simulink library "marlo_lib_v01"  (Simulink 8.1)
settings: Solver=ode45  StartTime=0.0  StopTime=10.0  RelTol=1e-3
undefined symbols (not defined in the file or in its folder): A_deriv_encoder, A_deriv_IMU, ANOMALY_INIT, B_deriv_encoder, B_deriv_IMU, C_deriv_encoder, C_deriv_IMU, CalibrationParams, Com1, D_deriv_encoder, D_deriv_IMU, Dt_deriv_encoder, Dt_deriv_IMU, EncoderAngleLimits, EncoderThreshold, IMUAngleLimits, IMUParams, IMUThreshold, KVHOrientationCal, m_XR17D15x, MAX_ANOMALY, MotorParams, none, standard, x0_deriv_encoder, x0_deriv_IMU, XOFF, XON
libraries: xpcethercatlib x307, speedgoatlib x26, xpcseriallib x15, simulink x8, marlo_lib_v01 x6, dspswit3 x2, xpclib x1
(part 5 of 6)

== system marlo_lib_v01/DAQ_WITH_SAFETY_IMU/DAQ/SerialIMU/TPMC466 ==
  In1 : Inport
  In2 : Inport  Port=2
  In3 : Inport  Port=3
  In4 : Inport  Port=4
  Board Setup : speedgoatlib/IO503/TEWS TPMC466 Internal blocks/Board Setup  irqnum=9  slot=brdslot
  "Enable TX " : speedgoatlib/IO503/TEWS TPMC466 Internal blocks/Enable TX   port=1  slot=brdslot
  Enable TX 1 : speedgoatlib/IO503/TEWS TPMC466 Internal blocks/Enable TX   port=2  slot=brdslot
  Enable TX 2 : speedgoatlib/IO503/TEWS TPMC466 Internal blocks/Enable TX   port=3  slot=brdslot
  Enable TX 3 : speedgoatlib/IO503/TEWS TPMC466 Internal blocks/Enable TX   port=4  slot=brdslot
  FIFO write 1 : xpcseriallib/FIFO write   size=1024  inputtype=8 bit uint null terminated  present=on  sampletime=-1  id=XMT channel 1, IRQ 9
  FIFO write 2 : xpcseriallib/FIFO write   size=1024  inputtype=8 bit uint null terminated  present=on  sampletime=-1  id=XMT channel 2, IRQ 9
  FIFO write 3 : xpcseriallib/FIFO write   size=1024  inputtype=8 bit uint null terminated  present=on  sampletime=-1  id=XMT channel 3, IRQ 9
  FIFO write 4 : xpcseriallib/FIFO write   size=1024  inputtype=8 bit uint null terminated  present=on  sampletime=-1  id=XMT channel 4, IRQ 9
  IRQ Source : xpclib/Asynchronous Event/IRQ Source  irqNo=9  preempt=off  b_type=None/Other  slot=brdslot
  RS232 ISR : Subsystem  TreatAsAtomicUnit=on  mask(RS232 ISR){slot=brdslot}
      mask help:
      | PMC521
      | Acromag
      | Interrupt Service Routine
      mask init:
      | subslot = slot;
      mask Display:
      | disp('PMC521\nAcromag\nISR');
      | port_label('input', 1, 'XMT1');
      | port_label('input', 2, 'XMT2');
      | port_label('input', 3, 'XMT3');
      | port_label('input', 4, 'XMT4');
      | port_label('input', 5, 'XMT5');
      | port_label('input', 6, 'XMT6');
      | port_label('input', 7, 'XMT7');
      | port_label('input', 8, 'XMT8');
      | port_label('output', 1, 'RCV1');
      | port_label('output', 2, 'RCV2');
      | port_label('output', 3, 'RCV3');
      | port_label('output', 4, 'RCV4');
      | port_label('output', 5, 'RCV5');
      | port_label('output', 6, 'RCV6');
      | port_label('output', 7, 'RCV7');
      | port_label('output', 8, 'RCV8');
  Rate Transition{,2,4..5} (4 alike) : RateTransition  Integrity=off  Deterministic=off
  Rate Transition{1,3,6..7} (4 alike) : RateTransition  Integrity=off  Deterministic=off  OutPortSampleTime=0
  Setup1 : speedgoatlib/IO503/TEWS TPMC466 Internal blocks/Setup   port=1  transceiver=RS422  standard=on  baudrate=921600  bauddivisor=1  mode8x=16x (standard)  prescale=off  width=8  nstop=1  parity=None  rlevel=quarter full (16)  ctsmode=none  xonoff=none  xon=17  xoff=19  rs485mode=off  rs485delay=1  slot=brdslot
  Setup2 : speedgoatlib/IO503/TEWS TPMC466 Internal blocks/Setup   port=2  transceiver=RS485 half-duplex  standard=on  baudrate=2764800  bauddivisor=1  mode8x=16x (standard)  prescale=off  width=8  nstop=1  parity=None  rlevel=quarter full (16)  ctsmode=none  xonoff=XON/XOFF  xon=17  xoff=19  rs485mode=on  rs485delay=1  slot=brdslot
  Setup3 : speedgoatlib/IO503/TEWS TPMC466 Internal blocks/Setup   port=3  transceiver=RS485 half-duplex  standard=on  baudrate=115200  bauddivisor=1  mode8x=16x (standard)  prescale=off  width=8  nstop=1  parity=None  rlevel=half full (32)  ctsmode=none  xonoff=none  xon=17  xoff=19  rs485mode=off  rs485delay=0  slot=brdslot
  Setup4 : speedgoatlib/IO503/TEWS TPMC466 Internal blocks/Setup   port=4  transceiver=RS485 half-duplex  standard=on  baudrate=115200  bauddivisor=1  mode8x=16x (standard)  prescale=off  width=8  nstop=1  parity=None  rlevel=half full (32)  ctsmode=none  xonoff=none  xon=17  xoff=19  rs485mode=off  rs485delay=0  slot=brdslot
  Out1 : Outport
  Out2 : Outport  Port=2
  Out3 : Outport  Port=3
  Out4 : Outport  Port=4
  wires:
  FIFO write 2/2 -> Enable TX 1/1
  In2/1 -> FIFO write 2/1
  FIFO write 2/1 -> Rate Transition2/1
  In1/1 -> FIFO write 1/1
  FIFO write 1/1 -> Rate Transition/1
  RS232 ISR/2(Recv 2) -> Rate Transition3/1
  RS232 ISR/1(Recv 1) -> Rate Transition1/1
  IRQ Source/1 -> RS232 ISR/Trigger
  FIFO write 1/2 -> "Enable TX "/1
  Rate Transition2/1 -> RS232 ISR/2(Xmt 2)
  Rate Transition/1 -> RS232 ISR/1(Xmt 1)
  Rate Transition3/1 -> Out2/1
  Rate Transition1/1 -> Out1/1
  FIFO write 3/2 -> Enable TX 2/1
  In3/1 -> FIFO write 3/1
  FIFO write 3/1 -> Rate Transition4/1
  FIFO write 4/2 -> Enable TX 3/1
  In4/1 -> FIFO write 4/1
  FIFO write 4/1 -> Rate Transition5/1
  Rate Transition4/1 -> RS232 ISR/3(Xmt 3)
  Rate Transition5/1 -> RS232 ISR/4(Xmt 4)
  Rate Transition6/1 -> Out3/1
  Rate Transition7/1 -> Out4/1
  RS232 ISR/3(Recv 3) -> Rate Transition6/1
  RS232 ISR/4(Recv 4) -> Rate Transition7/1

== system marlo_lib_v01/DAQ_WITH_SAFETY_IMU/DAQ/SerialIMU/UpdateOrientation ==
  FIFO : Inport
  Reset : Inport  Port=2
  Zero : Inport  Port=3
  Assignment : Assignment  IndexOptions=Index vector (port)  Indices=1  OutputSizes=1
  Compare To Constant1 : simulink/Logic and Bit Operations/Compare To Constant  relop===  const=1  OutDataTypeStr=uint8
  EstimateOrientation : MATLAB Function  TreatAsAtomicUnit=on
  "FIFO bin read " : xpcseriallib/FIFO bin read   header={char([254 129 255 85])}  lengths=[36]  hold=Zero output if no new data  enable=off  maxsize=36  outputtype=8 bit uint null terminated  sampletime=-1
  For Iterator : ForIterator
  MATLAB Function : MATLAB Function  TreatAsAtomicUnit=on
  Product : Product  RndMeth=Zero
  Unit Delay : UnitDelay  InitialCondition=[0; 0; 0]  SampleTime=-1
  Unit Delay1 : UnitDelay  InitialCondition=zeros(3,3)  SampleTime=-1
  Unit Delay2 : UnitDelay  InitialCondition=[0; 0; 0]  SampleTime=-1
  Unit Delay3 : UnitDelay  SampleTime=-1
  Rk : Outport  InitialOutput=zeros(3,3)
  wk : Outport  Port=2  InitialOutput=zeros(3,1)
  DeltaAngle : Outport  Port=3  InitialOutput=zeros(3,1)
  Acceleration : Outport  Port=4  InitialOutput=zeros(3,1)
  Status : Outport  Port=5  InitialOutput=0
  Sequence : Outport  Port=6  InitialOutput=[0; 0; 0; 0; 0]
  Temperature : Outport  Port=7  InitialOutput=0
  Valid : Outport  Port=8  InitialOutput=0
  wires:
  Unit Delay2/1 -> EstimateOrientation/7(wkm1)
  EstimateOrientation/2(wk) -> Unit Delay2/1, wk/1
  For Iterator/1 -> [Iter]
  Zero/1 -> Assignment/1
  Assignment/1 -> Sequence/1
  [Iter] -> Assignment/3
  "FIFO bin read "/1 -> MATLAB Function/1(P)
  Reset/1 -> [Reset]
  Unit Delay3/1 -> EstimateOrientation/9(Seqkm1)
  EstimateOrientation/4(Seqk) -> Unit Delay3/1
  FIFO/1 -> "FIFO bin read "/1
  Compare To Constant1/1 -> Product/2
  Product/1 -> EstimateOrientation/3(Status)
  [Reset] -> EstimateOrientation/5(Reset)
  Unit Delay1/1 -> EstimateOrientation/6(Rkm1)
  EstimateOrientation/1(Rk) -> Unit Delay1/1, Rk/1
  Unit Delay/1 -> EstimateOrientation/8(Akm1)
  EstimateOrientation/3(Ak) -> Unit Delay/1
  MATLAB Function/6(Valid) -> Compare To Constant1/1, Valid/1
  MATLAB Function/5(Temperature) -> Temperature/1
  MATLAB Function/4(Sequence) -> EstimateOrientation/4(Sequence), Assignment/2
  MATLAB Function/3(Status) -> Product/1, Status/1
  MATLAB Function/1(Rotation) -> EstimateOrientation/1(DeltaAngle), DeltaAngle/1
  MATLAB Function/2(Acceleration) -> EstimateOrientation/2(Acceleration), Acceleration/1

== system marlo_lib_v01/DAQ_WITH_SAFETY_IMU/DAQ/SerialIMU/TPMC466/RS232 ISR ==
  Xmt 1 : Inport
  Xmt 2 : Inport  Port=2
  Xmt 3 : Inport  Port=3
  Xmt 4 : Inport  Port=4
  function : TriggerPort  TriggerType=function-call
  While Iterator Subsystem : Subsystem  TreatAsAtomicUnit=on
  Recv 1 : Outport  SourceOfInitialOutputValue=Input signal
  Recv 2 : Outport  Port=2  SourceOfInitialOutputValue=Input signal
  Recv 3 : Outport  Port=3  SourceOfInitialOutputValue=Input signal
  Recv 4 : Outport  Port=4  SourceOfInitialOutputValue=Input signal
  wires:
  Xmt 1/1 -> While Iterator Subsystem/1(Xmt 1)
  Xmt 2/1 -> While Iterator Subsystem/2(Xmt 2)
  While Iterator Subsystem/1(Recv 1) -> Recv 1/1
  While Iterator Subsystem/2(Recv 2) -> Recv 2/1
  Xmt 3/1 -> While Iterator Subsystem/3(Xmt 3)
  Xmt 4/1 -> While Iterator Subsystem/4(Xmt 4)
  While Iterator Subsystem/3(Recv 3) -> Recv 3/1
  While Iterator Subsystem/4(Recv 4) -> Recv 4/1

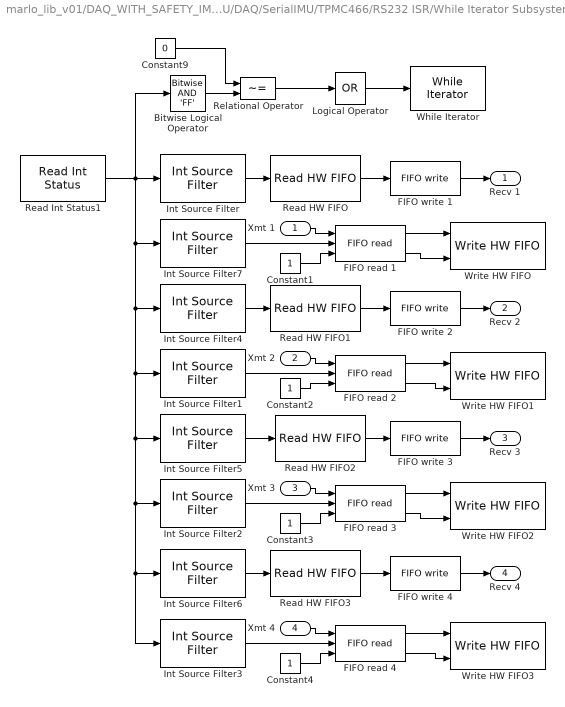
== system marlo_lib_v01/DAQ_WITH_SAFETY_IMU/DAQ/SerialIMU/TPMC466/RS232 ISR/While Iterator Subsystem ==
  Xmt 1 : Inport
  Xmt 2 : Inport  Port=2
  Xmt 3 : Inport  Port=3
  Xmt 4 : Inport  Port=4
  Bitwise Logical Operator : simulink/Logic and Bit Operations/Bitwise Operator  logicop=AND  UseBitMask=on  BitMask='FF'  BitMaskRealWorld=Stored Integer
  Constant{1..4} (4 alike) : Constant  OutDataTypeStr=uint32
  Constant9 : Constant  Value=0  OutDataTypeStr=uint32
  FIFO read {1..4} (4 alike) : xpcseriallib/FIFO read   maxsize=60  minsize=1  usedelimiter=off  delimiter=13  outputtype=count+32 bit uint  enable=on  enableout=on  sampletime=-1
  FIFO write 1 : xpcseriallib/FIFO write   size=1024  inputtype=count+32 bit uint  present=off  sampletime=-1  id=RCV channel 1, IRQ 9
  FIFO write 2 : xpcseriallib/FIFO write   size=1024  inputtype=count+32 bit uint  present=off  sampletime=-1  id=RCV channel 2, IRQ 9
  FIFO write 3 : xpcseriallib/FIFO write   size=1024  inputtype=count+32 bit uint  present=off  sampletime=-1  id=RCV channel 3, IRQ 9
  FIFO write 4 : xpcseriallib/FIFO write   size=1024  inputtype=count+32 bit uint  present=off  sampletime=-1  id=RCV channel 4, IRQ 9
  Int Source Filter : speedgoatlib/IO503/TEWS TPMC466 Internal blocks/Int Source Filter  port=1  value=Receive data
  Int Source Filter1 : speedgoatlib/IO503/TEWS TPMC466 Internal blocks/Int Source Filter  port=2  value=Transmitter empty
  Int Source Filter2 : speedgoatlib/IO503/TEWS TPMC466 Internal blocks/Int Source Filter  port=3  value=Transmitter empty
  Int Source Filter3 : speedgoatlib/IO503/TEWS TPMC466 Internal blocks/Int Source Filter  port=4  value=Transmitter empty
  Int Source Filter4 : speedgoatlib/IO503/TEWS TPMC466 Internal blocks/Int Source Filter  port=2  value=Receive data
  Int Source Filter5 : speedgoatlib/IO503/TEWS TPMC466 Internal blocks/Int Source Filter  port=3  value=Receive data
  Int Source Filter6 : speedgoatlib/IO503/TEWS TPMC466 Internal blocks/Int Source Filter  port=4  value=Receive data
  Int Source Filter7 : speedgoatlib/IO503/TEWS TPMC466 Internal blocks/Int Source Filter  port=1  value=Transmitter empty
  Logical Operator : Logic  Operator=OR  Inputs=1  AllPortsSameDT=off
  Read HW FIFO : speedgoatlib/IO503/TEWS TPMC466 Internal blocks/Read HW FIFO  port=1  flush=on  slot=subslot
  Read HW FIFO1 : speedgoatlib/IO503/TEWS TPMC466 Internal blocks/Read HW FIFO  port=2  flush=on  slot=subslot
  Read HW FIFO2 : speedgoatlib/IO503/TEWS TPMC466 Internal blocks/Read HW FIFO  port=3  flush=on  slot=subslot
  Read HW FIFO3 : speedgoatlib/IO503/TEWS TPMC466 Internal blocks/Read HW FIFO  port=4  flush=on  slot=subslot
  Read Int Status1 : speedgoatlib/IO503/TEWS TPMC466 Internal blocks/Read Int Status  slot=subslot
  Relational Operator : RelationalOperator  Operator=~=
  While Iterator : WhileIterator  MaxIters=65  WhileBlockType=do-while
  Write HW FIFO : speedgoatlib/IO503/TEWS TPMC466 Internal blocks/Write HW FIFO  port=1  slot=subslot
  Write HW FIFO1 : speedgoatlib/IO503/TEWS TPMC466 Internal blocks/Write HW FIFO  port=2  slot=subslot
  Write HW FIFO2 : speedgoatlib/IO503/TEWS TPMC466 Internal blocks/Write HW FIFO  port=3  slot=subslot
  Write HW FIFO3 : speedgoatlib/IO503/TEWS TPMC466 Internal blocks/Write HW FIFO  port=4  slot=subslot
  Recv 1 : Outport  SourceOfInitialOutputValue=Input signal
  Recv 2 : Outport  Port=2  SourceOfInitialOutputValue=Input signal
  Recv 3 : Outport  Port=3  SourceOfInitialOutputValue=Input signal
  Recv 4 : Outport  Port=4  SourceOfInitialOutputValue=Input signal
  wires:
  Int Source Filter3/1 -> FIFO read 4/2
  Xmt 4/1 -> FIFO read 4/1
  FIFO read 4/1 -> Write HW FIFO3/1
  FIFO read 4/2 -> Write HW FIFO3/2
  Constant4/1 -> FIFO read 4/3
  Logical Operator/1 -> While Iterator/1
  Relational Operator/1 -> Logical Operator/1
  Bitwise Logical Operator/1 -> Relational Operator/2
  Constant9/1 -> Relational Operator/1
  Read Int Status1/1 -> Int Source Filter/1, Int Source Filter7/1, Int Source Filter4/1, Int Source Filter1/1, Int Source Filter5/1, Int Source Filter2/1, Int Source Filter3/1, Int Source Filter6/1, Bitwise Logical Operator/1
  Int Source Filter/1 -> Read HW FIFO/1
  FIFO write 1/1 -> Recv 1/1
  Read HW FIFO/1 -> FIFO write 1/1
  Int Source Filter7/1 -> FIFO read 1/2
  Xmt 1/1 -> FIFO read 1/1
  Int Source Filter4/1 -> Read HW FIFO1/1
  FIFO write 2/1 -> Recv 2/1
  Read HW FIFO1/1 -> FIFO write 2/1
  Int Source Filter1/1 -> FIFO read 2/2
  Xmt 2/1 -> FIFO read 2/1
  FIFO read 2/1 -> Write HW FIFO1/1
  FIFO read 1/1 -> Write HW FIFO/1
  FIFO read 1/2 -> Write HW FIFO/2
  FIFO read 2/2 -> Write HW FIFO1/2
  Constant1/1 -> FIFO read 1/3
  Constant2/1 -> FIFO read 2/3
  Int Source Filter2/1 -> FIFO read 3/2
  Xmt 3/1 -> FIFO read 3/1
  FIFO read 3/1 -> Write HW FIFO2/1
  FIFO read 3/2 -> Write HW FIFO2/2
  Constant3/1 -> FIFO read 3/3
  Int Source Filter5/1 -> Read HW FIFO2/1
  Int Source Filter6/1 -> Read HW FIFO3/1
  FIFO write 3/1 -> Recv 3/1
  Read HW FIFO2/1 -> FIFO write 3/1
  FIFO write 4/1 -> Recv 4/1
  Read HW FIFO3/1 -> FIFO write 4/1

== stateflow chart CheckAndFilterIMU/AnomalyDetection ==
  state Init
    en, du:
    q_clean = q;
    q_last = q;
    dq_last = dq;
    ErrorCount = 0;
  state Run
    state Error
      en: dq_last = dq; //dq is delayed to prevent algebraic loops
      en, du:
      ErrorCount++;
      q_clean = q_last + ErrorCount*dq_last*ANOMALY_DT;
    state Nominal
      en, du:
      q_clean = q;
      q_last = q;
      dq_last = dq;
      ErrorCount = 0;
    (default) -> Nominal
    Nominal -> Error : [check_error()]
    Error -> Nominal [order 2] : [!check_error()]
  (default) -> Init
  Init -> Run : [!Reset && after(ANOMALY_INIT, tick)]
  Run -> Init : [Reset]
  Error -> Init [order 1] : [ErrorCount>MAX_ANOMALY]
  data: err function_output boolean; q input double size=1; dq input double size=1; q_clean output double size=1; ErrorCount output double; MAX_ANOMALY parameter double size=1; q_last local double size=1; dq_last local double size=1; ANOMALY_INIT parameter double size=1; q_limits input double size=2; Threshold input double size=1; Reset input boolean size=1; ANOMALY_DT input double size=1
  function err = check_error:
    | function err = check_error
    |     %#codegen
    |     err = (q<q_limits(1)) || (q>q_limits(2)) || (abs(q - q_clean) > (ErrorCount+1)*Threshold); 
    | end

== matlab function DAQ_WITH_SAFETY/DAQ/ConvertAmpCurrent ==
  data: adc_value input double; measuredCurrent output double
function measuredCurrent = convert(adc_value)
    %#codegen

    measuredCurrent = (adc_value) * 60.0 / 8192;
end

== stateflow chart CheckAndFilterEncoder/AnomalyDetection ==
  state Init
    en, du:
    q_clean = q;
    q_last = q;
    dq_last = dq;
    ErrorCount = 0;
  state Run
    state Error
      en: dq_last = dq; //dq is delayed to prevent algebraic loops
      en, du:
      ErrorCount++;
      q_clean = q_last + ErrorCount*dq_last*ANOMALY_DT;
    state Nominal
      en, du:
      q_clean = q;
      q_last = q;
      dq_last = dq;
      Counter_last = Counter;
      ErrorCount = 0;
    state MissedPacket
      en, du:
      q_clean = q_last + dq_last*ANOMALY_DT;
      ErrorCount--;
    (default) -> Nominal
    Nominal -> MissedPacket [order 1] : [0 && Counter == Counter_last]
    MissedPacket -> Nominal
    Nominal -> Error [order 2] : [check_error()]
    Error -> Nominal [order 2] : [!check_error()]
  (default) -> Init
  Init -> Run : [!Reset && after(ANOMALY_INIT, tick)]
  Run -> Init : [Reset]
  Error -> Init [order 1] : [ErrorCount>MAX_ANOMALY]
  data: err function_output boolean; q input double size=1; dq input double size=1; Counter input double; q_clean output double size=1; ErrorCount output double; MAX_ANOMALY parameter double size=1; q_last local double size=1; dq_last local double size=1; ANOMALY_INIT parameter double size=1; q_limits input double size=2; Threshold input double size=1; Reset input boolean size=1; ANOMALY_DT input double size=1; Counter_last local double size=1
  function err = check_error:
    | function err = check_error
    |     %#codegen
    |     err = (q<q_limits(1)) || (q>q_limits(2)) ...
    |         || (abs(q - q_clean) > (ErrorCount+1)*Threshold);
    | end

== matlab function SerialIMU/MATLAB Function ==
  data: D input double; M output double; T output double; valid output double
function [M,T,valid] = parseOrientation(D)
    %#codegen
    CMD = hex2dec('c5');
    LEN = 43;
    
    valid = 0;
    if (D(1) == CMD(1))
        computedChecksum = mod(sum(D(1:LEN-2)),2^16);
        receivedChecksum = 2^8*D(LEN-1)+D(LEN);
        valid = double(receivedChecksum == computedChecksum);
    end
    M = parseSingle(D(2:LEN-6,:));
    T = parseUint32(D(LEN-5:LEN-2,:))/62500;
end
%{
function C = parseBytes(D, N)
    D = [parseSingle(D(1:end-4,:)); parseUint32(D(end-3:end,:))/62500];
    C = mat2cell(D,N);
end
%}
function S = parseSingle(D)
    % S = double(typecast(uint8(reshape(flipud(reshape(D,4,[])), [], 1)),'single'));
    Stmp1 = uint32(flipud(reshape(D,4,[])));
    Stmp2 = Stmp1(1,:) + 256*Stmp1(2,:) + 65536*Stmp1(3,:) + 16777216*Stmp1(4,:);
    Stmp3 = typecast(Stmp2,'single');
    S = double(Stmp3');
end

function S = parseUint32(D)
    %S = double(typecast(uint8(reshape(flipud(reshape(D,4,[])), [], 1)),'uint32'));
    Stmp1 = uint32(flipud(reshape(D,4,[])));
    Stmp2 = Stmp1(1,:) + 256*Stmp1(2,:) + 65536*Stmp1(3,:) + 16777216*Stmp1(4,:);
    S = double(Stmp2');
end

function S = parseUint16(D)
    S = zeros(size(D,1)/2, size(D,2));
    for k=1:size(D,2)
        S(:,k) = double(typecast(uint8(reshape(flipud(reshape(D(:,k),2,[])), [], 1)),'uint16'));
    end
end

function D = fromSingle(S)
    D = reshape(flipud(reshape(typecast(single(S), 'uint8'), 4, [])), [], 1);
end

function D = fromUint16(S)
    D = reshape(flipud(reshape(typecast(uint16(S), 'uint8'), 2, [])), [], 1);
end

== matlab function DAQ_WITH_SAFETY/DAQ/ConvertLogicVoltage ==
  data: adc_value input double; logicVoltage output double
function logicVoltage = convert(adc_value)
    %#codegen
    
    MEDULLA_ADC_MAX_VOLTS     = 2.70;
    MEDULLA_ADC_OFFSET_COUNTS = 172;
    
    logicVoltage = (adc_value - MEDULLA_ADC_OFFSET_COUNTS) * (MEDULLA_ADC_MAX_VOLTS/(4095.0))  * 6.0;
end

== matlab function DAQ_WITH_SAFETY/DAQ/ConvertMotorVoltage ==
  data: adc_value input double; motorVoltage output double
function motorVoltage = convert(adc_value)
    %#codegen
    
    MOTOR_VOLTAGE_C_OFFSET    = 1300.0;
    MOTOR_VOLTAGE_V_CAL       = 60.2;
    MOTOR_VOLTAGE_C_CAL       = 3600.0;
    
    motorVoltage = (adc_value - MOTOR_VOLTAGE_C_OFFSET)*MOTOR_VOLTAGE_V_CAL/(MOTOR_VOLTAGE_C_CAL-MOTOR_VOLTAGE_C_OFFSET);
end

== matlab function DAQ_WITH_SAFETY/DAQ/ConvertThermistors ==
  data: adc_value input double; temperature output double
function temperature = convert(adc_value)
    %#codegen
    
    MEDULLA_ADC_MAX_VOLTS     = 2.70;
    MEDULLA_ADC_OFFSET_COUNTS = 172;
    
    processedADCValue = (adc_value - MEDULLA_ADC_OFFSET_COUNTS) * (MEDULLA_ADC_MAX_VOLTS/(4095.0));
    temperature       = (1.0./( (1.0/298.15) + (1.0/3988.0)*log(4700.0./((3.26./processedADCValue) - 1.0)/10000))) - 273.15;
end

== matlab function SerialIMU/M_to_Euler ==
  data: M_WI input double; EulerAngles output double; IMUParams input double
function EulerAngles = fcn(M_WI, IMUParams)
    %#codegen
    EulerAngles = MtoEuler(M_WI, IMUParams);
end

== matlab function DAQ_WITH_SAFETY/DAQ/EncodeSwitches ==
  data: Switches input double; LimitSwitchesEncoded output double
function LimitSwitchesEncoded = EncodeSwitches(Switches)
    LimitSwitchesVec     = uint32(Switches);
    LimitSwitchesEncoded = double(EncodeSwitches(LimitSwitchesVec));
end

== matlab function DAQ_WITH_SAFETY_IMU/DAQ/ConvertAmpCurrent ==
  data: adc_value input double; measuredCurrent output double
function measuredCurrent = convert(adc_value)
    %#codegen

    measuredCurrent = (adc_value) * 60.0 / 8192;
end

== matlab function DAQ_WITH_SAFETY/DAQ/calibrate ==
  data: CalibrationParams input double; AbsEncoders input double; IncEncoders input double; IncEncodersPrev input double; AbsAngle output double; Reset input double; IncAngle output double; RolloverIn input double; Rollover output double; IncCalTickIn input double; IncCalTick output double
function [AbsAngle, IncAngle, Rollover, IncCalTick] = calibrate(CalibrationParams,AbsEncoders,IncEncoders,IncEncodersPrev,Reset,RolloverIn,IncCalTickIn)
    %#codegen
    [AbsAngle, IncAngle, Rollover, IncCalTick] = calibrateEncoders(CalibrationParams,AbsEncoders,IncEncoders,IncEncodersPrev,Reset,RolloverIn,IncCalTickIn);
end

== matlab function DAQ_WITH_SAFETY/DAQ/GeneralizedCoordinates ==
  data: EncoderAngles input double; EncoderVelocities input double; q_clean output double; IMUAngles input double; IMUVelocities input double; UseMotorIncEncoders input double; UseIMU input double; dq_clean output double; BoomAndIMU output double; IMUTorsoOffset input double; GearOffset input double; Reset input double
function [q_clean, dq_clean, BoomAndIMU] = coords(EncoderAngles, EncoderVelocities, IMUAngles, IMUVelocities, UseMotorIncEncoders, UseIMU, IMUTorsoOffset, GearOffset, Reset)
    %#codegen
    
    if (Reset)
        q_clean  = zeros(13,1);
        dq_clean = zeros(13,1);
    else 
        q_clean  = EncoderAngles([17:19 1:6 15 7:8 16]);
        dq_clean = EncoderVelocities([17:19 1:6 15 7:8 16]);
        
        q_clean([8:9 11:12]) = q_clean([8:9 11:12]) + GearOffset*pi/180;
        if (UseMotorIncEncoders)
            q_clean([8:9 11:12])  = EncoderAngles(11:14);
            dq_clean([8:9 11:12]) = EncoderVelocities(11:14);
        end
        
        if (UseIMU)
            q_clean(1:3)  = IMUAngles + [0; IMUTorsoOffset]*pi/180;
            dq_clean(1:3) = IMUVelocities;
        end
    end
    
    BoomAndIMU = [EncoderAngles(17:19); EncoderVelocities(17:19); IMUAngles; IMUVelocities];
end

== matlab function DAQ_WITH_SAFETY/DAQ/convert_mtr_current_to_pwm ==
  data: params input double; u input double; y output double; Reset input double
function y = convert_to_pwm(params,u,Reset)
%#codegen
%This function takes motor torque command inputs and outputs
%pwm commands (for the Medulla) in UMich convention

y = zeros(6,1);

if (Reset)
    return
end

%The inputs, which are commanded motor torques 
leg_motor_1R_torque_cmd = u(1);
leg_motor_2R_torque_cmd = u(2);
hip_motor_3R_torque_cmd = u(3);
leg_motor_1L_torque_cmd = u(4);
leg_motor_2L_torque_cmd = u(5);
hip_motor_3L_torque_cmd = u(6);

%Parameters determined experimentally at U Mich
UMich_LEFT_MOTOR_HIP_DIRECTION = params(1); %The direction for the left hip motor. (UMich convention)
UMich_RIGHT_MOTOR_HIP_DIRECTION = params(2); %The direction for the right hip motor. (UMich convention)

% The parameters, from http://code.google.com/p/atrias/source/browse/robot_definitions/
%From robot_invariant_defs.h
MTR_MAX_COUNT = params(3); %The maximum commanded amplifier value. This is the maximum value sent to the Medullas for the amplifier command.
%From biped2_variant_defs.h
MTR_MAX_TORQUE = params(4); %Maximum motor torque for scaling
MTR_HIP_MAX_TORQUE = params(5); %Maximum hip motor torque for scaling
%From leg3_definitions.h (corresponds to our left leg)
%(Note that A=shin and B=thigh for OSU convention)
LEG3_MOTOR_A_DIRECTION = params(6);
LEG3_MOTOR_B_DIRECTION = params(7);
%From leg4_definitions.h (corresponds to our right leg)
%(Note that A=shin and B=thigh for OSU convention)
LEG4_MOTOR_A_DIRECTION = params(8);
LEG4_MOTOR_B_DIRECTION = params(9);

leg_torque_to_pwm = MTR_MAX_COUNT/MTR_MAX_TORQUE;
hip_torque_to_pwm = MTR_MAX_COUNT/MTR_HIP_MAX_TORQUE;

%Convert leg_motor_1L_torque_cmd
leg_motor_1L_direction = LEG3_MOTOR_A_DIRECTION;
y(1) = motor_torque_to_pwm(leg_motor_1L_direction,leg_torque_to_pwm,leg_motor_1L_torque_cmd);

%Convert leg_motor_2L_torque_cmd
leg_motor_2L_direction = LEG3_MOTOR_B_DIRECTION;
y(2) = motor_torque_to_pwm(leg_motor_2L_direction,leg_torque_to_pwm,leg_motor_2L_torque_cmd);

%Convert leg_motor_1R_torque_cmd
leg_motor_1R_direction = LEG4_MOTOR_A_DIRECTION;
y(3) = motor_torque_to_pwm(leg_motor_1R_direction,leg_torque_to_pwm,leg_motor_1R_torque_cmd);

%Convert leg_motor_2R_torque_cmd
leg_motor_2R_direction = LEG4_MOTOR_B_DIRECTION;
y(4) = motor_torque_to_pwm(leg_motor_2R_direction,leg_torque_to_pwm,leg_motor_2R_torque_cmd);

%Convert hip_motor_3R_torque_cmd
hip_motor_3R_direction = UMich_RIGHT_MOTOR_HIP_DIRECTION; %Verified experimentally
y(5) = motor_torque_to_pwm(hip_motor_3R_direction,hip_torque_to_pwm,hip_motor_3R_torque_cmd);

%Convert hip_motor_3L_torque_cmd
hip_motor_3L_direction = UMich_LEFT_MOTOR_HIP_DIRECTION; %Verified experimentally
y(6) = motor_torque_to_pwm(hip_motor_3L_direction,hip_torque_to_pwm,hip_motor_3L_torque_cmd);

end

function motor_pwm = motor_torque_to_pwm(motor_direction,torque_to_pwm_const,motor_torque_cmd)
   motor_pwm = motor_direction*torque_to_pwm_const*motor_torque_cmd;
end

== matlab function DAQ_WITH_SAFETY/SAFETY ==
  data: MotorCurrentCommand input double; MotorCurrentCommandSafe output double; MedullaCommand input double; IMUCommand input double; q input double; dq input double; Switches input double; Thermistors input double; MedullaCommandSafe output double; IMUCommandSafe output double; SafetyStateOut output double; LogicVoltage input double; SafetyCountIn input double; SafetyCountOut output double
function [MotorCurrentCommandSafe, MedullaCommandSafe, IMUCommandSafe, SafetyStateOut, SafetyCountOut] = SafetyCheck(MotorCurrentCommand, MedullaCommand, IMUCommand, q, dq, Switches, Thermistors, LogicVoltage, SafetyCountIn)
    %#codegen
    
    % Checks DAQ inputs and outputs to ensure that the commands sent to the
    % robot and the state reported by the robot are okay. Any invalid
    % commands to the robot are discarded, and default (zero) commands are
    % send instead. The cause of the failure can be traced by logging the
    % SafetyStateOut output.
    %
    % SafetyStateOut is a double so that it can be logged efficiently in
    % the same array as the other outputs. However, we set individual bits
    % of the significand to encode various error states. Since the uint64
    % data type is not supported for code generation, we are limited to
    % using 32 bits of the significand. Thus the safety state should be an
    % integer in the range 0 to 2^32-1.
    
    % SAFE OUTPUTS
    % THESE OUTPUTS ARE USED IN A HARD SHUTDOWN, AND CAUSE ALL COMMANDED
    % CURRENTS TO BE ZEROED AND THE MEDULLAS TO ENTER THE HALT STATE.
    MotorCurrentCommandSafe   = [0; 0; 0; 0; 0; 0];
    MedullaCommandSafe        = 4; % 4=HALT
    IMUCommandSafe            = 0;
    SafetyState               = uint32(0);
    
    % HARD SAFETY PARAMETERS
    % THE FOLLOWING PARAMETERS SPECIFY LIMITS WHICH, WHEN EXCEEDED, CAUSE
    % THE SAFETY TO LOCK DOWN THE ROBOT BY SENDING THE DEFAULT SAFE OUTPUTS
    % ABOVE.
    MAX_MOTOR_TEMP         = 80; % C
    MAX_MOTOR_CURRENT      = 120;  % Amps 
    VALID_MEDULLA_COMMANDS = [0 1 2 3 4 5 6 7];
    %VALID_IMU_COMMANDS     = [0 1 2]; % Meaningless for now
    
    MAX_TORSO_PITCH         = 35; % degrees
    MAX_TORSO_ROLL          = 20; % degrees
    MAX_LEG_ANGLE_DEVIATION = 40; % degrees from 180
    MAX_KNEE_ANGLE          = 80; % degrees; mechanical limit is 160 degrees
    MIN_KNEE_ANGLE          = 14.5; %22.5; % degrees; mechanical limit is reported to be 34.5 degrees
    MAX_LEG_LINK_FLEXION    = 60; % degrees from 180; mechanical limit is 107.5 degrees
    MAX_LEG_LINK_EXTENSION  = 20; % degrees from 180; mechanical limit is 45 degrees 
    % END (HARD SAFETY PARAMETERS)
    
    % SOFT SAFETY PARAMETERS
    % THE FOLLOWING PARAMETERS SPECIFY LIMITS WHICH DO NOT CAUSE THE SAFETY
    % TO LOCK DOWN THE WHOLE ROBOT. INSTEAD, APPROPRIATE CURRENTS ARE
    % LIMITED TO PREVENT DRIVING THE MOTORS IN A MANNER THAT MIGHT CAUSE
    % DAMAGE
    MAX_HIP_ANGLE_SOFT           = 7; % degrees; mechanical limit is reported to be 20 degrees
    MIN_HIP_ANGLE_SOFT           = -15; % degrees; mechanical limit is reported to be -10 degrees 
    
    SOFT_LIMIT_WIDTH_HIP         = 4;  % degrees
    SOFT_LIMIT_UMAX_HIP          = 15; % Amps
    % END (SOFT SAFETY PARAMETERS)
    
    
    % SAFETY STATE DEFINITION
    SSMASK_INVALID_MOTOR_COMMAND   = uint32(1);
    SSMASK_INVALID_MEDULLA_COMMAND = uint32(2);
    SSMASK_INVALID_IMU_COMMAND     = uint32(4);
    SSMASK_BAD_CONFIGURATION       = uint32(8);
    SSMASK_OVERTEMP                = uint32(256);   % Each motor will set one bit of second byte
    SSMASK_LIMSWITCH               = uint32(65536); 
    
    %{
    % CHECK THERMISTORS    
    SafetyState = bitor(SafetyState, bitshift(SSMASK_OVERTEMP, 0)*uint32(any(Thermistors(1:6)  >MAX_MOTOR_TEMP)));
    SafetyState = bitor(SafetyState, bitshift(SSMASK_OVERTEMP, 1)*uint32(any(Thermistors(7:12) >MAX_MOTOR_TEMP)));
    SafetyState = bitor(SafetyState, bitshift(SSMASK_OVERTEMP, 2)*uint32(any(Thermistors(13:15)>MAX_MOTOR_TEMP)));
    SafetyState = bitor(SafetyState, bitshift(SSMASK_OVERTEMP, 3)*uint32(any(Thermistors(16:21)>MAX_MOTOR_TEMP)));
    SafetyState = bitor(SafetyState, bitshift(SSMASK_OVERTEMP, 4)*uint32(any(Thermistors(22:27)>MAX_MOTOR_TEMP)));
    SafetyState = bitor(SafetyState, bitshift(SSMASK_OVERTEMP, 5)*uint32(any(Thermistors(28:30)>MAX_MOTOR_TEMP)));
    %}
    
    %{
    % CHECK LIMIT SWITCHES
    SafetyState = bitor(SafetyState, bitshift(SSMASK_LIMSWITCH, 0)*uint32(any(Thermistors(1:6)  >MAX_MOTOR_TEMP)));
    SafetyState = bitor(SafetyState, bitshift(SSMASK_LIMSWITCH, 1)*uint32(any(Thermistors(7:12) >MAX_MOTOR_TEMP)));
    SafetyState = bitor(SafetyState, bitshift(SSMASK_LIMSWITCH, 2)*uint32(any(Thermistors(13:15)>MAX_MOTOR_TEMP)));
    SafetyState = bitor(SafetyState, bitshift(SSMASK_LIMSWITCH, 3)*uint32(any(Thermistors(16:21)>MAX_MOTOR_TEMP)));
    SafetyState = bitor(SafetyState, bitshift(SSMASK_LIMSWITCH, 4)*uint32(any(Thermistors(22:27)>MAX_MOTOR_TEMP)));
    SafetyState = bitor(SafetyState, bitshift(SSMASK_LIMSWITCH, 5)*uint32(any(Thermistors(28:30)>MAX_MOTOR_TEMP)));
    %}
    
    % VALIDATE MOTOR COMMAND
    if any(~isfinite(MotorCurrentCommand)) ...                    % Check for NaN and +Inf and -Inf
            || any(abs(MotorCurrentCommand) > MAX_MOTOR_CURRENT)  % Check for extremely large commands
        
        SafetyState = bitor(SafetyState, SSMASK_INVALID_MOTOR_COMMAND);
    end
    
    % VALIDATE MEDULLA COMMAND
    if any(~ismember(MedullaCommand, VALID_MEDULLA_COMMANDS))
        SafetyState = bitor(SafetyState, SSMASK_INVALID_MEDULLA_COMMAND);
    end
    
    % VALIDATE IMU COMMAND
    %if any(~ismember(IMUCommand, VALID_IMU_COMMANDS))
    %    SafetyState = bitor(SafetyState, SSMASK_INVALID_IMU_COMMAND);
    %end
    
    
    % CHECK ROBOT CONFIGURATION (HARD SAFETY)   

    % THE FOLLOWING LIMITS, WHEN EXCEEDED, CAUSE THE SAFETY TO LOCK DOWN
    % THE ROBOT BY SENDING THE DEFAULT SAFE OUTPUTS ABOVE.
    qyT = q(2);
    qxT = q(3);
    qLA = [0 0 0 0.5 0.5   0   0 0 0 0 0 0 0; ...
           0 0 0   0   0 0.5 0.5 0 0 0 0 0 0]*q;
	qKA = [0 0 0  -1   1   0   0 0 0 0 0 0 0; ...
           0 0 0   0   0  -1   1 0 0 0 0 0 0]*q;
    qLegLinkFlexion = [0 0 0  -1   0   0   0 0 0 0 0 0 0; ...
                       0 0 0   0   1   0   0 0 0 0 0 0 0; ...
                       0 0 0   0   0  -1   0 0 0 0 0 0 0
                       0 0 0   0   0   0   1 0 0 0 0 0 0]*q + [1; -1; 1; -1]*pi;
                   
    if abs(qxT) > MAX_TORSO_PITCH*pi/180 ...
            || abs(qyT) > MAX_TORSO_ROLL*pi/180 ...
            || any(abs(qLA-pi) > MAX_LEG_ANGLE_DEVIATION*pi/180) ...
            || any(qKA > MAX_KNEE_ANGLE*pi/180) ...
            || any(qKA < MIN_KNEE_ANGLE*pi/180) ...
            || any(qLegLinkFlexion > MAX_LEG_LINK_FLEXION*pi/180) ...
            || any(qLegLinkFlexion < -MAX_LEG_LINK_EXTENSION*pi/180)
        
        SafetyState = bitor(SafetyState, SSMASK_BAD_CONFIGURATION);
    end
        
    
    % CHECK ROBOT CONFIGURATION (SOFT SAFETY)
    
    % THE FOLLOWING LIMITS, WHEN EXCEEDED, DO *NOT* CAUSE THE SAFETY TO
    % LOCK DOWN THE WHOLE ROBOT. INSTEAD, APPROPRIATE CURENTS ARE LIMITED
    % TO PREVENT DRIVING THE MOTORS IN A MANNER THAT MIGHT CAUSE DAMAGE
    
    %{
    % BGB 2014-05-21
    q3R = q(10);
    q3L = q(13);
    
    MotorCurrentCommand(3) = continuouslySaturate(MotorCurrentCommand(3), q3R, [MIN_HIP_ANGLE_SOFT MAX_HIP_ANGLE_SOFT]*pi/180, SOFT_LIMIT_WIDTH_HIP*pi/180, SOFT_LIMIT_UMAX_HIP);
    MotorCurrentCommand(6) = continuouslySaturate(MotorCurrentCommand(6), q3L, [MIN_HIP_ANGLE_SOFT MAX_HIP_ANGLE_SOFT]*pi/180, SOFT_LIMIT_WIDTH_HIP*pi/180, SOFT_LIMIT_UMAX_HIP);
    % END BGB 2014-05-21
    %}
    
    % The SafetyState output must be a double for efficient storage in an array with other DAQ outputs
    SafetyStateOut = double(SafetyState); 
    
    % IF EVERYTHING LOOKS OKAY (SAFETYSTATE==0), THEN PASS THE COMMANDS TO THE DAQ
    if (SafetyState==0)
        SafetyCountOut = max(0, SafetyCountIn-1);
    else
        SafetyCountOut = min(SafetyCountIn+1, 10);
    end
    
    if (SafetyCountOut<4)
        MotorCurrentCommandSafe = MotorCurrentCommand;
        MedullaCommandSafe = MedullaCommand;
        IMUCommandSafe = IMUCommand;
    end
end

== matlab function DAQ_WITH_SAFETY_IMU/DAQ/ConvertLogicVoltage ==
  data: adc_value input double; logicVoltage output double
function logicVoltage = convert(adc_value)
    %#codegen
    
    MEDULLA_ADC_MAX_VOLTS     = 2.70;
    MEDULLA_ADC_OFFSET_COUNTS = 172;
    
    logicVoltage = (adc_value - MEDULLA_ADC_OFFSET_COUNTS) * (MEDULLA_ADC_MAX_VOLTS/(4095.0))  * 6.0;
end

== matlab function DAQ_WITH_SAFETY_IMU/DAQ/ConvertMotorVoltage ==
  data: adc_value input double; motorVoltage output double
function motorVoltage = convert(adc_value)
    %#codegen
    
    MOTOR_VOLTAGE_C_OFFSET    = 1300.0;
    MOTOR_VOLTAGE_V_CAL       = 60.2;
    MOTOR_VOLTAGE_C_CAL       = 3600.0;
    
    motorVoltage = (adc_value - MOTOR_VOLTAGE_C_OFFSET)*MOTOR_VOLTAGE_V_CAL/(MOTOR_VOLTAGE_C_CAL-MOTOR_VOLTAGE_C_OFFSET);
end

== matlab function DAQ_WITH_SAFETY_IMU/DAQ/ConvertThermistors ==
  data: Temperatures output double; adc_value input double
function Temperatures  = convert(adc_value)
    %#codegen
    MEDULLA_ADC_MAX_VOLTS     = 2.70;
    MEDULLA_ADC_OFFSET_COUNTS = 172;
    
    processedADCValue = (adc_value - MEDULLA_ADC_OFFSET_COUNTS) * (MEDULLA_ADC_MAX_VOLTS/(4095.0));
    Temperatures      = (1.0./( (1.0/298.15) + (1.0/3988.0)*log(4700.0./((3.26./processedADCValue) - 1.0)/10000))) - 273.15;
end

== matlab function DAQ_WITH_SAFETY_IMU/DAQ/EncodeSwitches ==
  data: Switches input double; LimitSwitchesEncoded output double
function LimitSwitchesEncoded = EncodeSwitches(Switches)
    LimitSwitchesVec     = uint32(Switches);
    LimitSwitchesEncoded = double(EncodeSwitches(LimitSwitchesVec));
end

== matlab function DAQ_WITH_SAFETY_IMU/DAQ/GeneralizedCoordinates ==
  data: EncoderAngles input double; EncoderVelocities input double; q_clean output double; IMUAngles input double; IMUVelocities input double; UseMotorIncEncoders input double; UseIMU input double; dq_clean output double; BoomAndIMU output double; IMUTorsoOffset input double; GearOffset input double; Reset input double
function [q_clean, dq_clean, BoomAndIMU] = coords(EncoderAngles, EncoderVelocities, IMUAngles, IMUVelocities, UseMotorIncEncoders, UseIMU, IMUTorsoOffset, GearOffset, Reset)
    %#codegen
    
    if (Reset)
        q_clean  = zeros(13,1);
        dq_clean = zeros(13,1);
    else 
        q_clean  = EncoderAngles([17:19 1:6 15 7:8 16]);
        dq_clean = EncoderVelocities([17:19 1:6 15 7:8 16]);
        
        q_clean([8:9 11:12]) = q_clean([8:9 11:12]) + GearOffset*pi/180;
        if (UseMotorIncEncoders)
            q_clean([8:9 11:12])  = EncoderAngles(11:14);
            dq_clean([8:9 11:12]) = EncoderVelocities(11:14);
        end
        
        if (UseIMU)
            q_clean(1:3)  = IMUAngles + [0; IMUTorsoOffset]*pi/180;
            dq_clean(1:3) = IMUVelocities;
        end
    end
    
    BoomAndIMU = [EncoderAngles(17:19); EncoderVelocities(17:19); IMUAngles; IMUVelocities];
end

== matlab function DAQ_WITH_SAFETY_IMU/DAQ/MuxTemperatures ==
  data: t input double; Temperatures input double; TemperatureMuxed output double
function TemperatureMuxed  = convert(t, Temperatures)
    %#codegen
    k = mod(1000*t,100)+1;
    if (k>=1 && k<=30)
        TemperatureMuxed = Temperatures(k);
    elseif (k>30 && k<=40)
        TemperatureMuxed = k;
    else
        TemperatureMuxed = 0;
    end
end

== matlab function DAQ_WITH_SAFETY_IMU/DAQ/SerialIMU/ComputeEulerAngles ==
  data: RkIn input double; wk input double; RCal input double; Reset input double; R0In input double; ZYX output double; dZYX output double; Rk output double; R0 output double; YawRolloverIn input double; YawRollover output double
function [ZYX, dZYX, Rk, R0, YawRollover] = fcn(RkIn, wk, RCal, Reset, R0In, YawRolloverIn) %#codegen
    % Convert from IMU frame to robot frame and compute Euler angles. The
    % yaw angle is zeroed whenever (Reset) is true.
        
    if (Reset)
        % Compute the rotation matrix which zeroes the initial yaw
        qT0 = M_to_ZYX(RkIn*RCal);
        R0  = Rz(-qT0(1));
    else
        R0 = R0In;
    end
    
    % Transform from IMU to robot frame and zero initial yaw
    Rk = R0*RkIn*RCal;
    
    % Convert Rk to ZYX Euler angles
    ZYX = M_to_ZYX(Rk);
    
    % Unroll yaw
    YawRolloverCount = YawRolloverIn(1);
    PreviousYaw      = YawRolloverIn(2);
    CurrentYaw       = ZYX(1);
    YawRolloverCount = YawRolloverCount + getYawRollover(CurrentYaw, PreviousYaw);
    YawRollover      = [YawRolloverCount; CurrentYaw];
    ZYX(1)           = ZYX(1) + 2*pi*YawRolloverCount;
    
    % Compute Euler angle derivatives
    qzT = ZYX(1);
    qyT = ZYX(2);
    
    if cos(qyT)>1e-3
        dZYX = [0 -sin(qzT) cos(qzT)*cos(qyT); 0 cos(qzT) sin(qzT)*cos(qyT); 1 0 -sin(qyT)]\(R0*RkIn*wk);
    else
        dZYX = [0; 0; 0];
    end
end

function R = Rz(t)
    R = [cos(t) -sin(t) 0; sin(t) cos(t) 0; 0 0 1];
end

function Rollover = getYawRollover(CurrentYaw, PreviousYaw)
    % Determine if a rollover has occurred on yaw angle If a rollover is
    % detected, the output Rollover is either +1 or -1, depending on the
    % direction of the rollover.
  
    if (PreviousYaw>0 && CurrentYaw < (PreviousYaw-pi))
        Rollover = 1;
    elseif (PreviousYaw<0 && CurrentYaw > (PreviousYaw+pi))
        Rollover = -1;
    else
        Rollover = 0;
    end
end

== matlab function DAQ_WITH_SAFETY_IMU/DAQ/SerialIMU/UpdateOrientation/EstimateOrientation ==
  data: DeltaAngle input double; Acceleration input double; Status input double; Sequence input double; Reset input double; Rk output double; wk output double; Rkm1 input double; wkm1 input double; Akm1 input double; Ak output double; Seqkm1 input double; Seqk output double
function [Rk, wk, Ak, Seqk] = fcn(DeltaAngle,Acceleration,Status,Sequence,Reset,Rkm1,wkm1,Akm1,Seqkm1) %#codegen
    [Rk, wk, Ak, Seqk] = estimateOrientation(DeltaAngle,Acceleration,Rkm1,wkm1,Akm1,Status,Sequence,Seqkm1,Reset);
end

== matlab function DAQ_WITH_SAFETY_IMU/DAQ/SerialIMU/UpdateOrientation/MATLAB Function ==
  data: P input double; Rotation output double; Acceleration output double; Status output double; Sequence output double; Temperature output double; Valid output double
function [Rotation,Acceleration,Status,Sequence,Temperature,Valid] = KVHParsePacket(P)
    %#codegen
    CMD = [254; 129; 255; 85]; %hex2dec(['FE';'81';'FF';'55']);
    
    Valid = false;
    if all(P(1:4) == CMD)
        Valid = kvhCheckCRC(P(1:36));
    end
    
    Rotation = parseSingle(P(5:16,:));
    Acceleration = parseSingle(P(17:28,:));
    Status = double(P(29));
    Sequence = double(P(30));
    Temperature = parseInt16(P(31:32));
end

function S = parseSingle(D)
    Stmp1 = uint32(reshape(D,4,[]));
    Stmp2 = 16777216*Stmp1(1,:) + 65536*Stmp1(2,:) + 256*Stmp1(3,:) + Stmp1(4,:);
    Stmp3 = typecast(Stmp2,'single');
    S = double(Stmp3');
end

function S = parseInt16(D)
    Stmp1 = uint16(reshape(D,2,[]));
    Stmp2 = 256*Stmp1(1,:) + Stmp1(2,:);
    S = double(Stmp2');
end

== matlab function DAQ_WITH_SAFETY_IMU/DAQ/calibrate ==
  data: CalibrationParams input double; AbsEncoders input double; IncEncoders input double; IncEncodersPrev input double; AbsAngle output double; Reset input double; IncAngle output double; RolloverIn input double; Rollover output double; IncCalTickIn input double; IncCalTick output double
function [AbsAngle, IncAngle, Rollover, IncCalTick] = calibrate(CalibrationParams,AbsEncoders,IncEncoders,IncEncodersPrev,Reset,RolloverIn,IncCalTickIn)
    %#codegen
    [AbsAngle, IncAngle, Rollover, IncCalTick] = calibrateEncoders(CalibrationParams,AbsEncoders,IncEncoders,IncEncodersPrev,Reset,RolloverIn,IncCalTickIn);
end

== matlab function DAQ_WITH_SAFETY_IMU/DAQ/convert_mtr_current_to_pwm ==
  data: params input double; u input double; y output double; Reset input double
function y = convert_to_pwm(params,u,Reset)
%#codegen
%This function takes motor torque command inputs and outputs
%pwm commands (for the Medulla) in UMich convention

y = zeros(6,1);

if (Reset)
    return
end

%The inputs, which are commanded motor torques 
leg_motor_1R_torque_cmd = u(1);
leg_motor_2R_torque_cmd = u(2);
hip_motor_3R_torque_cmd = u(3);
leg_motor_1L_torque_cmd = u(4);
leg_motor_2L_torque_cmd = u(5);
hip_motor_3L_torque_cmd = u(6);

%Parameters determined experimentally at U Mich
UMich_LEFT_MOTOR_HIP_DIRECTION = params(1); %The direction for the left hip motor. (UMich convention)
UMich_RIGHT_MOTOR_HIP_DIRECTION = params(2); %The direction for the right hip motor. (UMich convention)

% The parameters, from http://code.google.com/p/atrias/source/browse/robot_definitions/
%From robot_invariant_defs.h
MTR_MAX_COUNT = params(3); %The maximum commanded amplifier value. This is the maximum value sent to the Medullas for the amplifier command.
%From biped2_variant_defs.h
MTR_MAX_TORQUE = params(4); %Maximum motor torque for scaling
MTR_HIP_MAX_TORQUE = params(5); %Maximum hip motor torque for scaling
%From leg3_definitions.h (corresponds to our left leg)
%(Note that A=shin and B=thigh for OSU convention)
LEG3_MOTOR_A_DIRECTION = params(6);
LEG3_MOTOR_B_DIRECTION = params(7);
%From leg4_definitions.h (corresponds to our right leg)
%(Note that A=shin and B=thigh for OSU convention)
LEG4_MOTOR_A_DIRECTION = params(8);
LEG4_MOTOR_B_DIRECTION = params(9);

leg_torque_to_pwm = MTR_MAX_COUNT/MTR_MAX_TORQUE;
hip_torque_to_pwm = MTR_MAX_COUNT/MTR_HIP_MAX_TORQUE;

%Convert leg_motor_1L_torque_cmd
leg_motor_1L_direction = LEG3_MOTOR_A_DIRECTION;
y(1) = motor_torque_to_pwm(leg_motor_1L_direction,leg_torque_to_pwm,leg_motor_1L_torque_cmd);

%Convert leg_motor_2L_torque_cmd
leg_motor_2L_direction = LEG3_MOTOR_B_DIRECTION;
y(2) = motor_torque_to_pwm(leg_motor_2L_direction,leg_torque_to_pwm,leg_motor_2L_torque_cmd);

%Convert leg_motor_1R_torque_cmd
leg_motor_1R_direction = LEG4_MOTOR_A_DIRECTION;
y(3) = motor_torque_to_pwm(leg_motor_1R_direction,leg_torque_to_pwm,leg_motor_1R_torque_cmd);

%Convert leg_motor_2R_torque_cmd
leg_motor_2R_direction = LEG4_MOTOR_B_DIRECTION;
y(4) = motor_torque_to_pwm(leg_motor_2R_direction,leg_torque_to_pwm,leg_motor_2R_torque_cmd);

%Convert hip_motor_3R_torque_cmd
hip_motor_3R_direction = UMich_RIGHT_MOTOR_HIP_DIRECTION; %Verified experimentally
y(5) = motor_torque_to_pwm(hip_motor_3R_direction,hip_torque_to_pwm,hip_motor_3R_torque_cmd);

%Convert hip_motor_3L_torque_cmd
hip_motor_3L_direction = UMich_LEFT_MOTOR_HIP_DIRECTION; %Verified experimentally
y(6) = motor_torque_to_pwm(hip_motor_3L_direction,hip_torque_to_pwm,hip_motor_3L_torque_cmd);

end

function motor_pwm = motor_torque_to_pwm(motor_direction,torque_to_pwm_const,motor_torque_cmd)
   motor_pwm = motor_direction*torque_to_pwm_const*motor_torque_cmd;
end
